simulink library "MapleSim_v142IE_400"  (R2020a)
settings: Solver=VariableStepAuto  StartTime=0.0  StopTime=10.0  RelTol=1e-3
Description:
  | Created by MapleSim.
settings Model: Creator=MapleSim  LastModifiedBy=BEDNASA

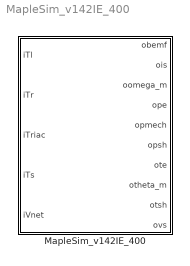
== system MapleSim_v142IE_400 ==
  MapleSim_v142IE_400 : Subsystem  Description=Subsystem: MapleSim_v142IE_400  mask(v142IE_400){ic=[22., 0.], Par1=.13e-3, Par2=.157, Par3=.4, Par4=.25e-5, Par5=0., Par6=.135, Par7=.5e-1, Par8=1., Par9=8.3, Par10=22., Par11=.8e-2, Par12=22., Par13=.386982e-2, Par14=.386982e-2, Par15=-1., Par16=0., Par17=.5, Par18=1., Par19=1., Par20=1., Par21=1., Par22=.1e-4, Par23=.1e-4, Par24=.8, Par25=293.15, Par26=293.15, Par27=22., ExtData=, MinStep=1/40}
      mask prompts: ic "Initial Conditions:"; Par1 "SP_v142_1_D:"; Par2 "SP_v142_1_Flux_f1m:"; Par3 "SP_v142_1_Flux_sa_max:"; Par4 "SP_v142_1_J:"; Par5 "SP_v142_1_Jadd:"; Par6 "SP_v142_1_Ls0:"; Par7 "SP_v142_1_Lsmin:"; Par8 "SP_v142_1_NPP:"; Par9 "SP_v142_1_Rs0:"; Par10 "SP_v142_1_TrRef:"; Par11 "SP_v142_1_Trp:"; Par12 "SP_v142_1_TsRef:"; Par13 "SP_v142_1_alpha_s:"; Par14 "SP_v142_1_d_magnet:"; Par15 "SP_v142_1_gain_k:"; Par16 "SP_v142_1_omega_m_start:"; Par17 "SP_v142_1_realToBoolean_threshold:"; Par18 "SP_v142_1_sPPMSM_UFSC_MBD_triac_v1_4_2_firstOrder_T:"; Par19 "SP_v142_1_sPPMSM_UFSC_MBD_triac_v1_4_2_firstOrder_k:"; Par20 "SP_v142_1_sPPMSM_UFSC_MBD_triac_v1_4_2_firstOrder1_T:"; Par21 "SP_v142_1_sPPMSM_UFSC_MBD_triac_v1_4_2_firstOrder1_k:"; Par22 "SP_v142_1_sPPMSM_UFSC_MBD_triac_v1_4_2_idealTriac_Snubberless_Goff:"; Par23 "SP_v142_1_sPPMSM_UFSC_MBD_triac_v1_4_2_idealTriac_Snubberless_Ron:"; Par24 "SP_v142_1_sPPMSM_UFSC_MBD_triac_v1_4_2_idealTriac_Snubberless_Vknee:"; Par25 "SP_v142_1_sPPMSM_UFSC_MBD_triac_v1_4_2_idealTriac_Snubberless_idealThyristor_T:"; Par26 "SP_v142_1_sPPMSM_UFSC_MBD_triac_v1_4_2_idealTriac_Snubberless_idealThyristor1_T:"; Par27 "SP_v142_1_theta_m_0:"; ExtData "Extended Visualization Data - File Name (leave blank to disable):"; MinStep "Extended Visualization Data - Minimum Sample Step:"
      mask help:
      | Variable Definitions
      |
      | Variable(s) in the Initial Condition Vector:
      |      x[ 3] = `Main.SP_PMSM.SP_v142_1.sPPMSM_UFSC_MBD_triac_v1_4_2.sPPMSM_UFSC_MBD_IO_v1_4_2.theta_m`(t)
      |      x[ 4] = diff(`Main.SP_PMSM.SP_v142_1.sPPMSM_UFSC_MBD_triac_v1_4_2.sPPMSM_UFSC_MBD_IO_v1_4_2.theta_m`(t),t)
      |
      | Variable(s) in the Output Vector:
      |    obemf:
      |      y[ 0] = `Main.SP_PMSM.obemf`(t)
      |    ois:
      |      y[ 1] = `Main.SP_PMSM.ois`(t)
      |    oomega_m:
      |      y[ 2] = `Main.SP_PMSM.oomega_m`(t)
      |    ope:
      |      y[ 3] = `Main.SP_PMSM.ope`(t)
      |    opmech:
      |      y[ 4] = `Main.SP_PMSM.opmech`(t)
      |    opsh:
      |      y[ 5] = `Main.SP_PMSM.opsh`(t)
      |    ote:
      |      y[ 6] = `Main.SP_PMSM.ote`(t)
      |    otheta_m:
      |      y[ 7] = `Main.SP_PMSM.otheta_m`(t)
      |    otsh:
      |      y[ 8] = `Main.SP_PMSM.otsh`(t)
      |    ovs:
      |      y[ 9] = `Main.SP_PMSM.ovs`(t)
      |
      | Variable(s) in the Input Vector:
      |    iTl:
      |      y[ 0] = `Main.SP_PMSM.iTl`(t)
      |    iTr:
      |      y[ 1] = `Main.SP_PMSM.iTr`(t)
      |    iTriac:
      |      y[ 2] = `Main.SP_PMSM.iTriac`(t)
      |    iTs:
      |      y[ 3] = `Main.SP_PMSM.iTs`(t)
      |    iVnet:
      |      y[ 4] = `Main.SP_PMSM.iVnet`(t)
      |
      | Parameter(s):
      |      p[ 0] = `Main.SP_PMSM.SP_v142_1.D` (default = .13e-3)
      |      p[ 1] = `Main.SP_PMSM.SP_v142_1.Flux_f1m` (default = .157)
      |      p[ 2] = `Main.SP_PMSM.SP_v142_1.Flux_sa_max` (default = .4)
      |      p[ 3] = `Main.SP_PMSM.SP_v142_1.J` (default = .25e-5)
      |      p[ 4] = `Main.SP_PMSM.SP_v142_1.Jadd` (default = 0.)
      |      p[ 5] = `Main.SP_PMSM.SP_v142_1.Ls0` (default = .135)
      |      p[ 6] = `Main.SP_PMSM.SP_v142_1.Lsmin` (default = .5e-1)
      |      p[ 7] = `Main.SP_PMSM.SP_v142_1.NPP` (default = 1., type = integer)
      |      p[ 8] = `Main.SP_PMSM.SP_v142_1.Rs0` (default = 8.3)
      |      p[ 9] = `Main.SP_PMSM.SP_v142_1.TrRef` (default = 22.)
      |      p[10] = `Main.SP_PMSM.SP_v142_1.Trp` (default = .8e-2)
      |      p[11] = `Main.SP_PMSM.SP_v142_1.TsRef` (default = 22.)
      |      p[12] = `Main.SP_PMSM.SP_v142_1.alpha_s` (default = .386982e-2)
      |      p[13] = `Main.SP_PMSM.SP_v142_1.d_magnet` (default = .386982e-2)
      |      p[14] = `Main.SP_PMSM.SP_v142_1.gain.k` (default = -1.)
      |      p[15] = `Main.SP_PMSM.SP_v142_1.omega_m_start` (default = 0.)
      |      p[16] = `Main.SP_PMSM.SP_v142_1.realToBoolean.threshold` (default = .5)
      |      p[17] = `Main.SP_PMSM.SP_v142_1.sPPMSM_UFSC_MBD_triac_v1_4_2.firstOrder.T` (default = 1.)
      |      p[18] = `Main.SP_PMSM.SP_v142_1.sPPMSM_UFSC_MBD_triac_v1_4_2.firstOrder.k` (default = 1.)
      |      p[19] = `Main.SP_PMSM.SP_v142_1.sPPMSM_UFSC_MBD_triac_v1_4_2.firstOrder1.T` (default = 1.)
      |      p[20] = `Main.SP_PMSM.SP_v142_1.sPPMSM_UFSC_MBD_triac_v1_4_2.firstOrder1.k` (default = 1.)
      |      p[21] = `Main.SP_PMSM.SP_v142_1.sPPMSM_UFSC_MBD_triac_v1_4_2.idealTriac_Snubberless.Goff` (default = .1e-4)
      |      p[22] = `Main.SP_PMSM.SP_v142_1.sPPMSM_UFSC_MBD_triac_v1_4_2.idealTriac_Snubberless.Ron` (default = .1e-4)
      |      p[23] = `Main.SP_PMSM.SP_v142_1.sPPMSM_UFSC_MBD_triac_v1_4_2.idealTriac_Snubberless.Vknee` (default = .8)
      |      p[24] = `Main.SP_PMSM.SP_v142_1.sPPMSM_UFSC_MBD_triac_v1_4_2.idealTriac_Snubberless.idealThyristor.T` (default = 293.15)
      |      p[25] = `Main.SP_PMSM.SP_v142_1.sPPMSM_UFSC_MBD_triac_v1_4_2.idealTriac_Snubberless.idealThyristor1.T` (default = 293.15)
      |      p[26] = `Main.SP_PMSM.SP_v142_1.theta_m_0` (default = 22.)
      mask Help: <!DOCTYPE html PUBLIC "-//W3C//DTD HTML 4.01 Transitional//EN" "http://www.w3.org/TR/1999/REC-html401-19991224/loose.dtd"> <html lang="en"> <head> <title>MapleSim_v142IE_400 :: MapleSim model</title> <style type="text/css"> body { background-color: white; margin:10px;} h1 { color: #990000; font-size: x-large; } h2 { color: #990000; font-size: large; margin-top:0ex;     margin-bottom:0ex;   font-weight:bold;  } h3 { color:#990000;  margin-top:0ex;   margin-bottom:0ex;  font-weight:bold;    font-size: medium; } h4 { color:black;    margin-top:0ex;   margin-bottom:0ex;  font-weight:bold;    font-size: medium; } /* Vertical space in tables other than the header and footer banners */ table.body { margin-top: 2ex; margin-bottom: 2ex;} /* Make the text shrink to fit narrow windows, but not stretch too far in wide windows. */ p,h1,h2,div.content div { max-width: 600px; } pre.codeinput { background: #EEEEEE; padding: 10px;} @media print { pre.codeinput { word-wrap:break-word; width:100%; } } span.keyword { color: #0000FF} span.comment { color: #228B22} span.string { color: #A020F0} span.untermstring {color: #B20000} span.syscmd { color: #B28C00} pre.error { color: red;} p.footer { text-align: right; font-size: xx-small; font-weight: lighter; font-style: italic; color: gray; } </style> <meta name="generator" content="DocBook XSL Stylesheets V1.52.2"> <meta name="chunktype" content="refpage"> <meta http-equiv="Content-Script-Type" content="text/javascript"> </head> <body> <a name="top_of_page"></a> <p style="font-size:1px;"> <a name="f8-894621"></a> <a name="transferfcn"></a> <a class="indexterm" name="zmw57dd0e42758"></a></p> <h1 class="reftitle">MapleSim_v142IE_400</h1> <p>Simulink Block generated by MapleSim Connector</p> <p><a name="f8-894627"></a></p> <h1>Description <span class="inlinemediaobject"></span></h1> <p><a class="indexterm" name="zmw57dd0e42781"></a></p> <p>The v142IE_400 model runs in the continuous domain and is created in the MapleSim modeling environment. The discrete S-Function block MapleSim_v142IE_400 is created using MapleSim Connector. The block is a 5-input, 10-output, 27-parameter system.</p> <p><a name="f8-894641"></a></p> <h1>System Variables</h1> <p>The following variables are used in the S-Function block:</p>  State Variable(s)<dl><dd>x[ 0] = `Main.SP_PMSM.SP_v142_1.sPPMSM_UFSC_MBD_triac_v1_4_2.firstOrder.y`(t)   (*)</dd></br><dd>x[ 1] = `Main.SP_PMSM.SP_v142_1.sPPMSM_UFSC_MBD_triac_v1_4_2.firstOrder1.y`(t)   (*)</dd></br><dd>x[ 2] = `Main.SP_PMSM.SP_v142_1.sPPMSM_UFSC_MBD_triac_v1_4_2.sPPMSM_UFSC_MBD_IO_v1_4_2.Flux_sa`(t)   (*)</dd></br><dd>x[ 3] = `Main.SP_PMSM.SP_v142_1.sPPMSM_UFSC_MBD_triac_v1_4_2.sPPMSM_UFSC_MBD_IO_v1_4_2.theta_m`(t)</dd></br><dd>x[ 4] = diff(`Main.SP_PMSM.SP_v142_1.sPPMSM_UFSC_MBD_triac_v1_4_2.sPPMSM_UFSC_MBD_IO_v1_4_2.theta_m`(t),t)</dd></br></dl><p>(*) fixed initial condition due to initial equation</p> Output Variable(s)<dl><dd>obemf:</dd></br><dd>&nbsp;&nbsp;y[ 0] = `Main.SP_PMSM.obemf`(t)</dd></br><dd>ois:</dd></br><dd>&nbsp;&nbsp;y[ 1] = `Main.SP_PMSM.ois`(t)</dd></br><dd>oomega_m:</dd></br><dd>&nbsp;&nbsp;y[ 2] = `Main.SP_PMSM.oomega_m`(t)</dd></br><dd>ope:</dd></br><dd>&nbsp;&nbsp;y[ 3] = `Main.SP_PMSM.ope`(t)</dd></br><dd>opmech:</dd></br><dd>&nbsp;&nbsp;y[ 4] = `Main.SP_PMSM.opmech`(t)</dd></br><dd>opsh:</dd></br><dd>&nbsp;&nbsp;y[ 5] = `Main.SP_PMSM.opsh`(t)</dd></br><dd>ote:</dd></br><dd>&nbsp;&nbsp;y[ 6] = `Main.SP_PMSM.ote`(t)</dd></br><dd>otheta_m:</dd></br><dd>&nbsp;&nbsp;y[ 7] = `Main.SP_PMSM.otheta_m`(t)</dd></br><dd>otsh:</dd></br><dd>&nbsp;&nbsp;y[ 8] = `Main.SP_PMSM.otsh`(t)</dd></br><dd>ovs:</dd></br><dd>&nbsp;&nbsp;y[ 9] = `Main.SP_PMSM.ovs`(t)</dd></br></dl> Input Variable(s)<dl><dd>iTl:</dd></br><dd>&nbsp;&nbsp;y[ 0] = `Main.SP_PMSM.iTl`(t)</dd></br><dd>iTr:</dd></br><dd>&nbsp;&nbsp;y[ 1] = `Main.SP_PMSM.iTr`(t)</dd></br><dd>iTriac:</dd></br><dd>&nbsp;&nbsp;y[ 2] = `Main.SP_PMSM.iTriac`(t)</dd></br><dd>iTs:</dd></br><dd>&nbsp;&nbsp;y[ 3] = `Main.SP_PMSM.iTs`(t)</dd></br><dd>iVnet:</dd></br><dd>&nbsp;&nbsp;y[ 4] = `Main.SP_PMSM.iVnet`(t)</dd></br></dl> Parameter(s)<dl><dd>p[ 0] = `Main.SP_PMSM.SP_v142_1.D` (default = .13e-3)</dd></br><dd>p[ 1] = `Main.SP_PMSM.SP_v142_1.Flux_f1m` (default = .157)</dd></br><dd>p[ 2] = `Main.SP_PMSM.SP_v142_1.Flux_sa_max` (default = .4)</dd></br><dd>p[ 3] = `Main.SP_PMSM.SP_v142_1.J` (default = .25e-5)</dd></br><dd>p[ 4] = `Main.SP_PMSM.SP_v142_1.Jadd` (default = 0.)</dd></br><dd>p[ 5] = `Main.SP_PMSM.SP_v142_1.Ls0` (default = .135)</dd></br><dd>p[ 6] = `Main.SP_PMSM.SP_v142_1.Lsmin` (default = .5e-1)</dd></br><dd>p[ 7] = `Main.SP_PMSM.SP_v142_1.NPP` (default = 1., type = integer)</dd></br><dd>p[ 8] = `Main.SP_PMSM.SP_v142_1.Rs0` (default = 8.3)</dd></br><dd>p[ 9] = `Main.SP_PMSM.SP_v142_1.TrRef` (default = 22.)</dd></br><dd>p[10] = `Main.SP_PMSM.SP_v142_1.Trp` (default = .8e-2)</dd></br><dd>p[11] = `Main.SP_PMSM.SP_v142_1.TsRef` (default = 22.)</dd></br><dd>p[12] = `Main.SP_PMSM.SP_v142_1.alpha_s` (default = .386982e-2)</dd></br><dd>p[13] = `Main.SP_PMSM.SP_v142_1.d_magnet` (default = .386982e-2)</dd></br><dd>p[14] = `Main.SP_PMSM.SP_v142_1.gain.k` (default = -1.)</dd></br><dd>p[15] = `Main.SP_PMSM.SP_v142_1.omega_m_start` (default = 0.)</dd></br><dd>p[16] = `Main.SP_PMSM.SP_v142_1.realToBoolean.threshold` (default = .5)</dd></br><dd>p[17] = `Main.SP_PMSM.SP_v142_1.sPPMSM_UFSC_MBD_triac_v1_4_2.firstOrder.T` (default = 1.)</dd></br><dd>p[18] = `Main.SP_PMSM.SP_v142_1.sPPMSM_UFSC_MBD_triac_v1_4_2.firstOrder.k` (default = 1.)</dd></br><dd>p[19] = `Main.SP_PMSM.SP_v142_1.sPPMSM_UFSC_MBD_triac_v1_4_2.firstOrder1.T` (default = 1.)</dd></br><dd>p[20] = `Main.SP_PMSM.SP_v142_1.sPPMSM_UFSC_MBD_triac_v1_4_2.firstOrder1.k` (default = 1.)</dd></br><dd>p[21] = `Main.SP_PMSM.SP_v142_1.sPPMSM_UFSC_MBD_triac_v1_4_2.idealTriac_Snubberless.Goff` (default = .1e-4)</dd></br><dd>p[22] = `Main.SP_PMSM.SP_v142_1.sPPMSM_UFSC_MBD_triac_v1_4_2.idealTriac_Snubberless.Ron` (default = .1e-4)</dd></br><dd>p[23] = `Main.SP_PMSM.SP_v142_1.sPPMSM_UFSC_MBD_triac_v1_4_2.idealTriac_Snubberless.Vknee` (default = .8)</dd></br><dd>p[24] = `Main.SP_PMSM.SP_v142_1.sPPMSM_UFSC_MBD_triac_v1_4_2.idealTriac_Snubberless.idealThyristor.T` (default = 293.15)</dd></br><dd>p[25] = `Main.SP_PMSM.SP_v142_1.sPPMSM_UFSC_MBD_triac_v1_4_2.idealTriac_Snubberless.idealThyristor1.T` (default = 293.15)</dd></br><dd>p[26] = `Main.SP_PMSM.SP_v142_1.theta_m_0` (default = 22.)</dd></br></dl></p> <p><a name="f8-894651"></a></p><h1>Data Type Support</h1> <p>The MapleSim_v142IE_400 block accepts inputs and outputs signals of type <tt>double</tt>.</p> <a name="f8-894653"></a><h1>Parameters</h1><dl> <dt><a name="zmw57dd0e42948"></a><b><span class="term">Initial Condition</span>s</b></dt> <dd> <p>The row vector of initial conditions. A vector can be specified to initialize the state variables of the system.</p></dd> <dd> <p>The initial values of the following states are fixed based upon initial equations: x[ 0]x[ 1]x[ 2]</p></dd><dt><a name="zmw57dd0e42958"></a><span class="term"><b>Parameters</b></span></dt> <dd> <p>The scalars or the row vector of tunable parameters.</p></dd> </dl> <dt><a name="zmw57dd0e42968"></a> </dt><h1>Characteristics</h1> <table cellspacing="0" class="body" cellpadding="4" border="2"><colgroup><col width="41%"><col width="59%"></colgroup><tbody> <tr valign="top"><td bgcolor="#F2F2F2"><p>Direct Feedthrough</p></td><td bgcolor="#F2F2F2"><p>Yes, only if the block has no state variables.</p></td></tr> <tr valign="top"><td bgcolor="#F2F2F2"><p>Sample Time</p></td><td bgcolor="#F2F2F2"><p> Discrete</p></td></tr> <tr valign="top"><td bgcolor="#F2F2F2"><p>Scalar Expansion</p></td><td bgcolor="#F2F2F2"><p>No</p></td></tr> <tr valign="top"><td bgcolor="#F2F2F2"><p>State</p></td><td bgcolor="#F2F2F2"><p>Yes</p></td></tr> <tr valign="top"><td bgcolor="#F2F2F2"><p>Dimensionalized</p></td><td bgcolor="#F2F2F2"><p>Yes</p></td></tr> <tr valign="top"><td bgcolor="#F2F2F2"><p>Zero Crossing</p></td><td bgcolor="#F2F2F2"><p>Yes</p></td></tr> </tbody></table> <p></p><h1>Maple / MapleSim / MapleSim Connector Details</h1> <p></p><dd><p>Maple 2020.2, X86 64 WINDOWS, Nov 11 2020, Build ID 1502365</p></dd><dd><p>MapleSim 2020.2 Connector for FMI, Wed Nov 11 11:47:50 EST 2020, 1502365</p></dd><dd><p>GlobalOptimization 2020.0, Thu Mar  5 01:29:12 EST 2020, 1455132</p></dd><dd><p>MapleSim 2020.2, Wed Nov 11 11:47:02 EST 2020, 1502365</p></dd><dd><p>MapleSim 2020.2 Connector, Wed Nov 11 11:48:10 EST 2020, 1502365</p></dd><p></p></body></html>
      mask Display: color('blue');text(5,12,'Generated by MapleSim');

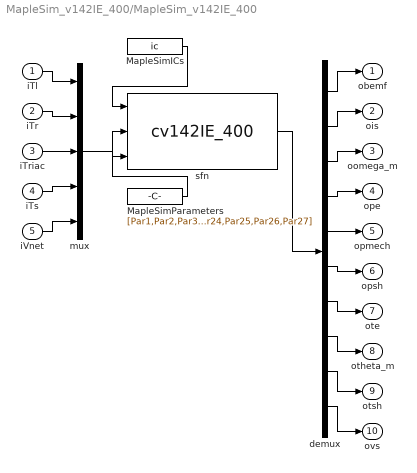
== system MapleSim_v142IE_400/MapleSim_v142IE_400 ==
  iTl : Inport
  iTr : Inport  Port=2
  iTriac : Inport  Port=3
  iTs : Inport  Port=4
  iVnet : Inport  Port=5
  MapleSimICs : Constant  Value=ic
  MapleSimParameters : Constant  Value=[Par1,Par2,Par3,Par4,Par5,Par6,Par7,Par8,Par9,Par10,Par11,Par12,Par13,Par14,Par15,Par16,Par17,Par18,Par19,Par20,Par21,Par22,Par23,Par24,Par25,Par26,Par27]
  demux : Demux  Outputs=[1 1 1 1 1 1 1 1 1 1]
  mux : Mux  Inputs=5
  sfn : S-Function  Description=Generated by MapleSim  FunctionName=cv142IE_400  Parameters=ExtData,MinStep  PortCounts=[3, 1]  SFunctionDeploymentMode=off  EnableBusSupport=off
  obemf : Outport
  ois : Outport  Port=2
  oomega_m : Outport  Port=3
  ope : Outport  Port=4
  opmech : Outport  Port=5
  opsh : Outport  Port=6
  ote : Outport  Port=7
  otheta_m : Outport  Port=8
  otsh : Outport  Port=9
  ovs : Outport  Port=10
  wires:
  MapleSimICs/1 -> sfn/1
  MapleSimParameters/1 -> sfn/2
  mux/1 -> sfn/3
  iTl/1 -> mux/1
  iTr/1 -> mux/2
  iTriac/1 -> mux/3
  iTs/1 -> mux/4
  iVnet/1 -> mux/5
  sfn/1 -> demux/1
  demux/1 -> obemf/1
  demux/2 -> ois/1
  demux/3 -> oomega_m/1
  demux/4 -> ope/1
  demux/5 -> opmech/1
  demux/6 -> opsh/1
  demux/7 -> ote/1
  demux/8 -> otheta_m/1
  demux/9 -> otsh/1
  demux/10 -> ovs/1
